simulink model "Rundenzeitsimulation"  (R2017a)
settings: Solver=VariableStepAuto  StartTime=0.0  StopTime=1  RelTol=1e-3
settings Model: Creator=alexa  LastModifiedBy=alexa

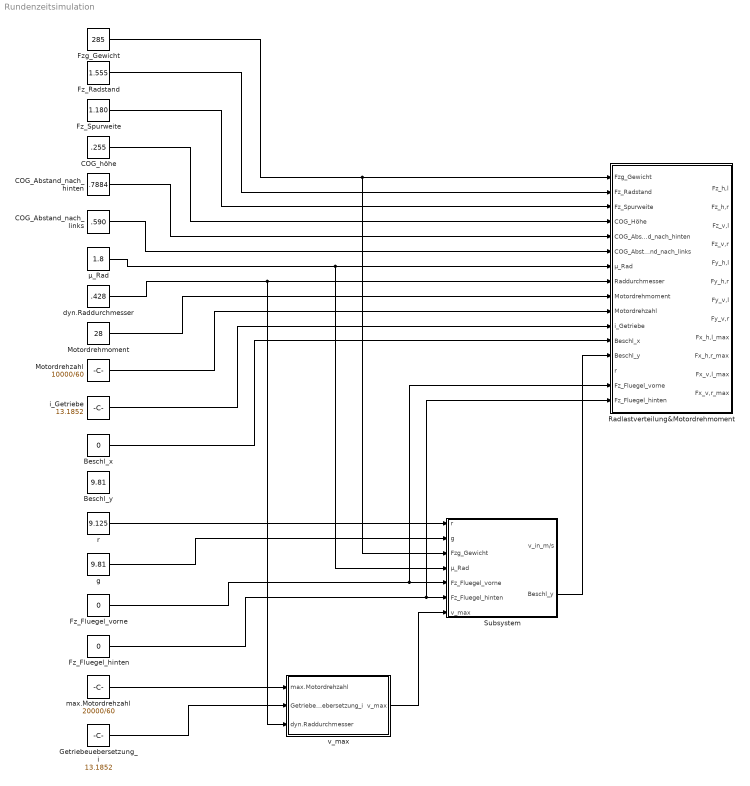
== system Rundenzeitsimulation ==
  Beschl_x : Constant  Value=0
  Beschl_y : Constant  Value=9.81
  COG_Abstand_nach_hinten : Constant  Value=.7884
  COG_Abstand_nach_links : Constant  Value=.590
  COG_höhe : Constant  Value=.255
  Fz_Fluegel_hinten : Constant  Value=0
  Fz_Fluegel_vorne : Constant  Value=0
  Fz_Radstand : Constant  Value=1.555
  Fz_Spurweite : Constant  Value=1.180
  Fzg_Gewicht : Constant  Value=285
  Getriebeuebersetzung_i : Constant  Value=13.1852
  Motordrehmoment : Constant  Value=28
  Motordrehzahl : Constant  Value=10000/60
  Radlastverteilung&Motordrehmoment : Subsystem  TreatAsAtomicUnit=on
  Subsystem : Subsystem
  dyn.Raddurchmesser : Constant  Value=.428
  g : Constant  Value=9.81
  i_Getriebe : Constant  Value=13.1852
  max.Motordrehzahl : Constant  Value=20000/60
  r : Constant  Value=9.125
  v_max : Subsystem
  μ_Rad : Constant  Value=1.8
  wires:
  Fzg_Gewicht/1 -> Subsystem/3(Fzg_Gewicht), Radlastverteilung&Motordrehmoment/1(Fzg_Gewicht)
  Fz_Radstand/1 -> Radlastverteilung&Motordrehmoment/2(Fz_Radstand)
  Fz_Spurweite/1 -> Radlastverteilung&Motordrehmoment/3(Fz_Spurweite)
  COG_höhe/1 -> Radlastverteilung&Motordrehmoment/4(COG_Höhe)
  COG_Abstand_nach_hinten/1 -> Radlastverteilung&Motordrehmoment/5(COG_Abstand_nach_hinten)
  COG_Abstand_nach_links/1 -> Radlastverteilung&Motordrehmoment/6(COG_Abstand_nach_links)
  μ_Rad/1 -> Subsystem/4(μ_Rad), Radlastverteilung&Motordrehmoment/7(μ_Rad)
  dyn.Raddurchmesser/1 -> v_max/3(dyn.Raddurchmesser), Radlastverteilung&Motordrehmoment/8(Raddurchmesser)
  Motordrehmoment/1 -> Radlastverteilung&Motordrehmoment/9(Motordrehmoment)
  Motordrehzahl/1 -> Radlastverteilung&Motordrehmoment/10(Motordrehzahl)
  i_Getriebe/1 -> Radlastverteilung&Motordrehmoment/11(i_Getriebe)
  Beschl_x/1 -> Radlastverteilung&Motordrehmoment/12(Beschl_x)
  Fz_Fluegel_vorne/1 -> Radlastverteilung&Motordrehmoment/15(Fz_Fluegel_vorne), Subsystem/5(Fz_Fluegel_vorne)
  g/1 -> Subsystem/2(g)
  r/1 -> Subsystem/1(r)
  Getriebeuebersetzung_i/1 -> v_max/2(Getriebeuebersetzung_i)
  max.Motordrehzahl/1 -> v_max/1(max.Motordrehzahl)
  v_max/1(v_max) -> Subsystem/7(v_max)
  Fz_Fluegel_hinten/1 -> Radlastverteilung&Motordrehmoment/16(Fz_Fluegel_hinten), Subsystem/6(Fz_Fluegel_hinten)
  Subsystem/2(Beschl_y) -> Radlastverteilung&Motordrehmoment/13(Beschl_y)

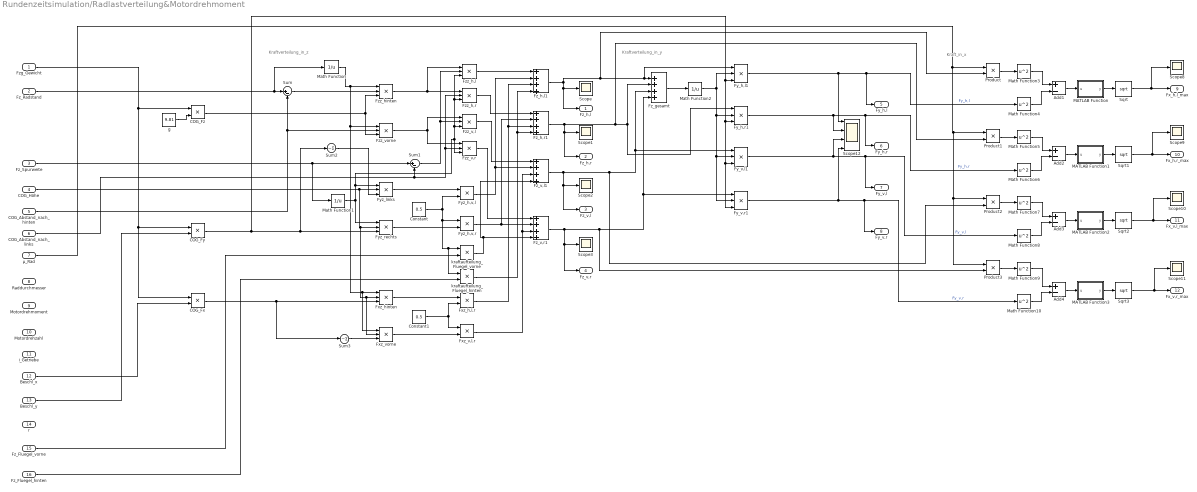
== system Rundenzeitsimulation/Radlastverteilung&Motordrehmoment ==
  note: Kraft_in_x
  note: Kraftverteilung_in_y
  note: Kraftverteilung_in_z
  Fzg_Gewicht : Inport
  Fz_Radstand : Inport  Port=2
  Fz_Spurweite : Inport  Port=3
  COG_Höhe : Inport  Port=4  Unit=mm
  COG_Abstand_nach_hinten : Inport  Port=5
  COG_Abstand_nach_links : Inport  Port=6
  μ_Rad : Inport  Port=7
  Raddurchmesser : Inport  Port=8
  Motordrehmoment : Inport  Port=9
  Motordrehzahl : Inport  Port=10
  i_Getriebe : Inport  Port=11
  Beschl_x : Inport  Port=12
  Beschl_y : Inport  Port=13
  r : Inport  Port=14
  Fz_Fluegel_vorne : Inport  Port=15
  Fz_Fluegel_hinten : Inport  Port=16
  Add{1..4} (4 alike) : Sum  Inputs=+-
  COG_Fx : Product
  COG_Fy : Product
  COG_Fz : Product
  Constant : Constant  Value=0.5
  Constant1 : Constant  Value=0.5
  Fxz_h,l,r : Product
  Fxz_hinten : Product  Inputs=3
  Fxz_v,l,r : Product
  Fxz_vorne : Product  Inputs=3
  Fy_h,l1 : Product  Inputs=3
  Fy_h,r1 : Product  Inputs=3
  Fy_v,l1 : Product  Inputs=3
  Fy_v,r1 : Product  Inputs=3
  Fyz_h,v,l : Product
  Fyz_h,v,r : Product
  Fyz_links : Product  Inputs=3
  Fyz_rechts : Product  Inputs=3
  Fz_gesamt : Sum  Inputs=4  OutMin=0
  Fz_h,l1 : Sum  Inputs=4  OutMin=0
  Fz_h,r1 : Sum  Inputs=4  OutMin=0
  Fz_v,l1 : Sum  Inputs=4  OutMin=0
  Fz_v,r1 : Sum  Inputs=4  OutMin=0
  Fzz_h,l : Product  Inputs=3
  Fzz_h,r : Product  Inputs=3
  Fzz_hinten : Product  Inputs=3
  Fzz_v,l : Product  Inputs=3
  Fzz_v,r : Product  Inputs=3
  Fzz_vorne : Product  Inputs=3
  MATLAB Function : MATLAB Function  TreatAsAtomicUnit=on
  MATLAB Function1 : MATLAB Function  TreatAsAtomicUnit=on
  MATLAB Function2 : MATLAB Function  TreatAsAtomicUnit=on
  MATLAB Function3 : MATLAB Function  TreatAsAtomicUnit=on
  Math Function : Math  Operator=reciprocal  SaturateOnIntegerOverflow=on
  Math Function1 : Math  Operator=reciprocal  SaturateOnIntegerOverflow=on
  Math Function{3..10} (8 alike) : Math  Operator=square  SaturateOnIntegerOverflow=on
  Math Function2 : Math  Operator=reciprocal  SaturateOnIntegerOverflow=on
  Product{,1..3} (4 alike) : Product
  Scope{,1..3,8..11} (8 alike) : Scope
  Scope12 : Scope  NumInputPorts=4
  Sqrt{,1..3} (4 alike) : Sqrt  SaturateOnIntegerOverflow=on
  Sum : Sum  Inputs=|+-
  Sum1 : Sum  Inputs=|+-
  Sum2 : Sum  Inputs=-
  Sum3 : Sum  Inputs=-
  g : Constant  Value=9.81
  kraftaufteilung_Fluegel_hinten : Product
  kraftaufteilung_Fluegel_vorne : Product
  Fz_h,l : Outport
  Fz_h,r : Outport  Port=2
  Fz_v,l : Outport  Port=3
  Fz_v,r : Outport  Port=4
  Fy_h,l : Outport  Port=5
  Fy_h,r : Outport  Port=6
  Fy_v,l : Outport  Port=7
  Fy_v,r : Outport  Port=8
  Fx_h,l_max : Outport  Port=9
  Fx_h,r_max : Outport  Port=10
  Fx_v,l_max : Outport  Port=11
  Fx_v,r_max : Outport  Port=12
  wires:
  Fzg_Gewicht/1 -> COG_Fy/1, COG_Fx/1, COG_Fz/1
  Beschl_x/1 -> COG_Fx/2
  g/1 -> COG_Fz/2
  Beschl_y/1 -> COG_Fy/2
  Fz_Spurweite/1 -> Sum1/1, Math Function1/1
  COG_Abstand_nach_links/1 -> Fzz_v,r/2, Fzz_h,r/2, Sum1/2
  Fz_Radstand/1 -> Math Function/1, Sum/1
  COG_Abstand_nach_hinten/1 -> Fzz_vorne/2, Sum/2
  Sum/1 -> Fzz_hinten/2
  COG_Fz/1 -> Fzz_hinten/3, Fzz_vorne/3
  COG_Fy/1 -> Fyz_rechts/3, Sum2/1, Fy_v,r1/3, Fy_v,l1/3, Fy_h,r1/3, Fy_h,l1/3
  COG_Höhe/1 -> Fxz_vorne/2, Fxz_hinten/2, Fyz_rechts/2, Fyz_links/2
  Sum2/1 -> Fyz_links/3
  Math Function/1 -> Fzz_hinten/1, Fzz_vorne/1, Fxz_hinten/1, Fxz_vorne/1
  COG_Fx/1 -> Fxz_hinten/3, Sum3/1
  Sum3/1 -> Fxz_vorne/3
  Fzz_hinten/1 -> Fzz_h,l/1, Fzz_h,r/1
  Fzz_vorne/1 -> Fzz_v,r/1, Fzz_v,l/1
  Sum1/1 -> Fzz_v,l/2, Fzz_h,l/2
  Math Function1/1 -> Fzz_v,r/3, Fzz_v,l/3, Fzz_h,r/3, Fzz_h,l/3, Fyz_links/1, Fyz_rechts/1
  Constant/1 -> kraftaufteilung_Fluegel_hinten/1, kraftaufteilung_Fluegel_vorne/1, Fyz_h,v,r/1, Fyz_h,v,l/2
  Fyz_rechts/1 -> Fyz_h,v,r/2
  Fyz_links/1 -> Fyz_h,v,l/1
  Fxz_vorne/1 -> Fxz_v,l,r/2
  Fxz_hinten/1 -> Fxz_h,l,r/1
  Constant1/1 -> Fxz_v,l,r/1, Fxz_h,l,r/2
  Fzz_h,r/1 -> Fz_h,r1/1
  Fzz_h,l/1 -> Fz_h,l1/1
  Fyz_h,v,l/1 -> Fz_h,l1/2, Fz_v,l1/2
  Fxz_h,l,r/1 -> Fz_h,l1/3, Fz_h,r1/3
  Fyz_h,v,r/1 -> Fz_v,r1/2, Fz_h,r1/2
  Fzz_v,l/1 -> Fz_v,l1/1
  Fxz_v,l,r/1 -> Fz_v,r1/3, Fz_v,l1/3
  Fzz_v,r/1 -> Fz_v,r1/1
  Fz_gesamt/1 -> Math Function2/1
  Math Function2/1 -> Fy_h,r1/2, Fy_v,r1/2, Fy_v,l1/2, Fy_h,l1/2
  Fy_h,l1/1 -> Scope12/1, Math Function4/1, Fy_h,l/1  "Fy_h,l"
  Fy_h,r1/1 -> Scope12/2, Fy_h,r/1, Math Function6/1  "Fy_h,r"
  Fy_v,l1/1 -> Scope12/3, Fy_v,l/1, Math Function8/1  "Fy_v,l"
  Fy_v,r1/1 -> Scope12/4, Fy_v,r/1, Math Function10/1  "Fy_v,r"
  Fz_Fluegel_vorne/1 -> kraftaufteilung_Fluegel_vorne/2
  Fz_Fluegel_hinten/1 -> kraftaufteilung_Fluegel_hinten/2
  kraftaufteilung_Fluegel_vorne/1 -> Fz_v,l1/4, Fz_v,r1/4
  kraftaufteilung_Fluegel_hinten/1 -> Fz_h,r1/4, Fz_h,l1/4
  μ_Rad/1 -> Product3/1, Product2/1, Product1/1, Product/1
  Fz_h,r1/1 -> Fz_h,r/1, Scope1/1, Fy_h,r1/1, Fz_gesamt/2, Product1/2
  Fz_v,r1/1 -> Product3/2, Fy_v,r1/1, Fz_gesamt/4, Scope3/1, Fz_v,r/1
  Fz_v,l1/1 -> Fy_v,l1/1, Fz_gesamt/3, Product2/2, Fz_v,l/1, Scope2/1
  Fz_h,l1/1 -> Product/2, Fy_h,l1/1, Fz_gesamt/1, Scope/1, Fz_h,l/1
  Product1/1 -> Math Function5/1
  Product3/1 -> Math Function9/1
  Product/1 -> Math Function3/1
  Add4/1 -> MATLAB Function3/1(u)
  Sqrt1/1 -> Scope9/1, Fx_h,r_max/1
  Add2/1 -> MATLAB Function1/1(u)
  Sqrt/1 -> Scope8/1, Fx_h,l_max/1
  Product2/1 -> Math Function7/1
  Add1/1 -> MATLAB Function/1(u)
  Sqrt2/1 -> Scope10/1, Fx_v,l_max/1
  Add3/1 -> MATLAB Function2/1(u)
  Math Function3/1 -> Add1/1
  Math Function4/1 -> Add1/2
  Math Function5/1 -> Add2/1
  Math Function6/1 -> Add2/2
  Math Function7/1 -> Add3/1
  Math Function8/1 -> Add3/2
  Math Function9/1 -> Add4/1
  Math Function10/1 -> Add4/2
  Sqrt3/1 -> Scope11/1, Fx_v,r_max/1
  MATLAB Function/1(y) -> Sqrt/1
  MATLAB Function1/1(y) -> Sqrt1/1
  MATLAB Function2/1(y) -> Sqrt2/1
  MATLAB Function3/1(y) -> Sqrt3/1

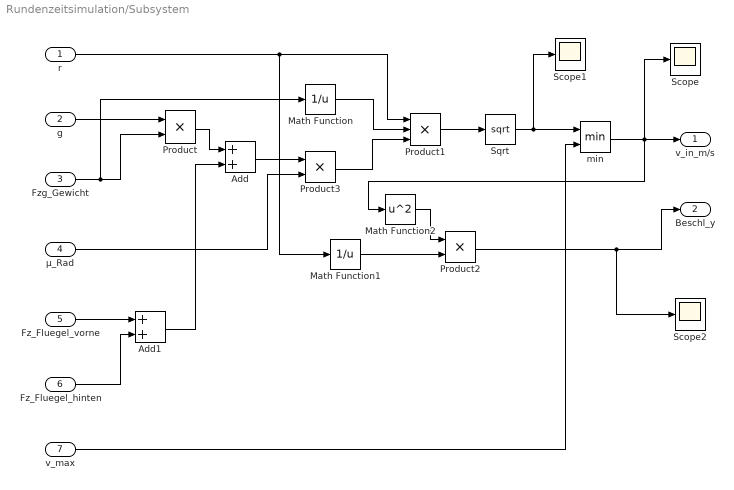
== system Rundenzeitsimulation/Subsystem ==
  r : Inport
  g : Inport  Port=2
  Fzg_Gewicht : Inport  Port=3
  μ_Rad : Inport  Port=4
  Fz_Fluegel_vorne : Inport  Port=5
  Fz_Fluegel_hinten : Inport  Port=6
  v_max : Inport  Port=7
  Add : Sum
  Add1 : Sum
  Math Function : Math  Operator=reciprocal  SaturateOnIntegerOverflow=on
  Math Function1 : Math  Operator=reciprocal  SaturateOnIntegerOverflow=on
  Math Function2 : Math  Operator=square  SaturateOnIntegerOverflow=on
  Product : Product
  Product1 : Product  Inputs=3
  Product2 : Product
  Product3 : Product
  Scope : Scope
  Scope1 : Scope
  Scope2 : Scope
  Sqrt : Sqrt  SaturateOnIntegerOverflow=on
  min : MinMax  Inputs=2
  v_in_m/s : Outport
  Beschl_y : Outport  Port=2
  wires:
  g/1 -> Product/1
  Fzg_Gewicht/1 -> Math Function/1, Product/2
  Product/1 -> Add/1
  Math Function/1 -> Product1/2
  r/1 -> Math Function1/1, Product1/1
  Product1/1 -> Sqrt/1
  Sqrt/1 -> Scope1/1, min/1
  v_max/1 -> min/2
  min/1 -> Math Function2/1, Scope/1, v_in_m/s/1
  Math Function1/1 -> Product2/2
  Product2/1 -> Scope2/1, Beschl_y/1
  Math Function2/1 -> Product2/1
  Fz_Fluegel_vorne/1 -> Add1/1
  Fz_Fluegel_hinten/1 -> Add1/2
  Add1/1 -> Add/2
  Product3/1 -> Product1/3
  Add/1 -> Product3/1
  μ_Rad/1 -> Product3/2

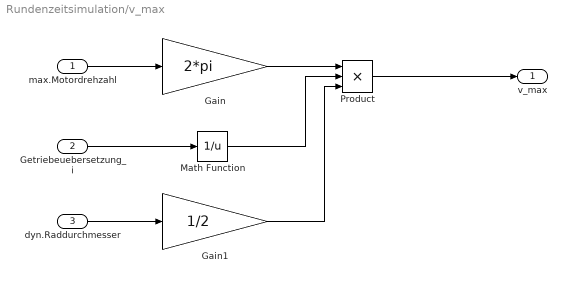
== system Rundenzeitsimulation/v_max ==
  max.Motordrehzahl : Inport
  Getriebeuebersetzung_i : Inport  Port=2
  dyn.Raddurchmesser : Inport  Port=3
  Gain : Gain  Gain=2*pi
  Gain1 : Gain  Gain=1/2
  Math Function : Math  Operator=reciprocal  SaturateOnIntegerOverflow=on
  Product : Product  Inputs=3
  v_max : Outport
  wires:
  max.Motordrehzahl/1 -> Gain/1
  Gain/1 -> Product/1
  Getriebeuebersetzung_i/1 -> Math Function/1
  Math Function/1 -> Product/2
  Product/1 -> v_max/1
  dyn.Raddurchmesser/1 -> Gain1/1
  Gain1/1 -> Product/3

== matlab function Rundenzeitsimulation/Radlastverteilung&Motordrehmoment/MATLAB Function1 ==
  data: u input; y output
function y = fcn(u)
if u>0
y = u;
else 
    y=0;
end

== matlab function Rundenzeitsimulation/Radlastverteilung&Motordrehmoment/MATLAB Function ==
  data: u input; y output
function y = fcn(u)
if u>0
y = u;
else 
    y=0;
end

== matlab function Rundenzeitsimulation/Radlastverteilung&Motordrehmoment/MATLAB Function2 ==
  data: u input; y output
function y = fcn(u)
if u>0
y = u;
else 
    y=0;
end

== matlab function Rundenzeitsimulation/Radlastverteilung&Motordrehmoment/MATLAB Function3 ==
  data: u input; y output
function y = fcn(u)
if u>0
y = u;
else 
    y=0;
end
